simulink model "EngineModel_scaled_27_7_2016_with_new_maps"  (R2021a)
settings: Solver=ode4  StartTime=0.0  StopTime=30  FixedStep=0.2  RelTol=1e-3  EnableMultiTasking=on
values from neighbouring files (symbols this model uses):
  Fanmap_2 = [1 1 1 1 1 1 1 1 1 1 275.724 325.4224 ... (330 elements, 10x3x11)]    [enginemaps2.mat]
  HPCompmap_2 = [1 1 1 1 1 1 1 1 1 1 32.390865 37.6623195 ... (330 elements, 10x3x11)]    [enginemaps2.mat]
  HPTurbinemap_2 = [0.24979968 0.24979968 0.24979968 0.24979968 0.24979968 0.24979968 0.24979968 0.24979968 0.24979968 0.24979968 0.004250667 0.005047667 ... (330 elements, 10x3x11)]    [enginemaps2.mat]
  LPCompmap_2 = [1 1 1 1 1 1 1 1 1 1 34.17260994 40.23277722 ... (330 elements, 10x3x11)]    [enginemaps2.mat]
  LPTurbinemap_2 = [0.665969797 0.665969797 0.665969797 0.665969797 0.665969797 0.665969797 0.665969797 0.665969797 0.00912 0.013173333 0.015706667 0.01672 ... (264 elements, 8x3x11)]    [enginemaps2.mat]
undefined symbols (not defined in the file or in its folder): Adiabatic_compression_fan, Adiabatic_compression_HPC, Adiabatic_compression_LPC, coldnozzle, compression_ram, cond_f2, D, datatables, hotnozzle, HPT1, if_Nth, if_Ntl, if_Z, LPT, performance1, thermo_combustor, turbo
libraries: dspmtrx3 x10, aerolibatmos2 x8, dspsigattribs x3, dspsolvers x2, dspfactors x1
(part 9 of 14)

== system EngineModel_scaled_27_7_2016_with_new_maps/Double spool TFE CF6-50 steady state modeling (BOING 747-200)/Error Due to Vs/Error Due To Dv7/HPT/ HP turbine ==
  Pt45 : Inport
  Cp45_old : Inport  Port=2
  F_A : Inport  Port=3
  Ht45_old : Inport  Port=4
  Wg4 : Inport  Port=5
  Wg45 : Inport  Port=6
  wach : Inport  Port=7
  Ht3 : Inport  Port=8
  Demux : Demux  Outputs=5
      settings: DisplayOption=none
  Interpreted MATLAB Function : MATLABFcn  MATLABFcn=turbo (u(1),u(2),u(3),u(4),u(5),u(6),u(7),u(8))  OutputDimensions=5
  Mux : Mux  Inputs=8
      settings: DisplayOption=signals
  Cp45 : Outport
  Tt45 : Outport  Port=2
  S45 : Outport  Port=3
  Ht45 : Outport  Port=4
  F/A : Outport  Port=5
  wires:
  Mux/1 -> Interpreted MATLAB Function/1
  Interpreted MATLAB Function/1 -> Demux/1
  Pt45/1 -> Mux/1
  Cp45_old/1 -> Mux/2
  F_A/1 -> Mux/3
  Ht45_old/1 -> Mux/4
  Wg4/1 -> Mux/5
  Wg45/1 -> Mux/6
  wach/1 -> Mux/7
  Ht3/1 -> Mux/8
  Demux/1 -> Cp45/1
  Demux/2 -> Tt45/1
  Demux/3 -> S45/1
  Demux/4 -> Ht45/1
  Demux/5 -> F/A/1

== system EngineModel_scaled_27_7_2016_with_new_maps/Double spool TFE CF6-50 steady state modeling (BOING 747-200)/Error Due to Vs/Error Due To Dv7/HPT/enthalpy_MAPS ==
  Ht4 : Inport
  Tt4 : Inport  Port=2
  Tt2.5 : Inport  Port=3
  Nch : Inport  Port=4
  TFth : Inport  Port=5
  " \"unit conversion\"" : Constant  Value=4.184
  Display{1..7} (7 alike) : Display
  HPT map : Subsystem
  Nch_Nth : Subsystem
  Product1 : Product  Inputs=*/  SaturateOnIntegerOverflow=on  OutDataTypeStr=Inherit: Same as first input
  Product5 : Product  Inputs=***  SaturateOnIntegerOverflow=on  OutDataTypeStr=Inherit: Same as first input
  Sum : Sum  Inputs=-+  SaturateOnIntegerOverflow=on
  Sum1 : Sum  Inputs=-+  SaturateOnIntegerOverflow=on
  Ht45s : Outport
  (DH/T)th : Outport  Port=2
  Ht45_old : Outport  Port=3
  wires:
  Sum1/1 -> Display4/1, Ht45s/1
  Nch/1 -> Nch_Nth/3(Nch)
  Nch_Nth/1(Nth) -> HPT map/1(Nth), Display5/1
  TFth/1 -> HPT map/2(TFth)
  HPT map/1((DH/T)th) -> Product5/3, Display1/1, (DH/T)th/1
  Ht4/1 -> Display3/1, Sum/2, Sum1/2
  Product5/1 -> Display2/1, Sum/1, Product1/1
  HPT map/2(etath) -> Display6/1, Product1/2
  Product1/1 -> Sum1/1
  Tt4/1 -> Product5/2, Nch_Nth/1(Tt4)
  Tt2.5/1 -> Nch_Nth/2(Tt2.5)
  " \"unit conversion\""/1 -> Product5/1
  Sum/1 -> Display7/1, Ht45_old/1

== system EngineModel_scaled_27_7_2016_with_new_maps/Double spool TFE CF6-50 steady state modeling (BOING 747-200)/Error Due to Vs/Error Due To Dv7/HPT/thermo_turbine ==
  Ht45s : Inport
  Ht45_old : Inport  Port=2
  Pt4 : Inport  Port=3
  Cp4 : Inport  Port=4
  F/A : Inport  Port=5
  S4 : Inport  Port=6
  Demux : Demux
      settings: DisplayOption=none
  Interpreted MATLAB Function : MATLABFcn  MATLABFcn=HPT1 (u(1),u(2),u(3),u(4),u(5),u(6))  OutputDimensions=4
  Mux : Mux  Inputs=6
      settings: DisplayOption=signals
  Pt45 : Outport
  Tt45 : Outport  Port=2
  S45 : Outport  Port=3
  Cp45 : Outport  Port=4
  wires:
  Interpreted MATLAB Function/1 -> Demux/1
  Mux/1 -> Interpreted MATLAB Function/1
  Ht45s/1 -> Mux/1
  Ht45_old/1 -> Mux/2
  Pt4/1 -> Mux/3
  Cp4/1 -> Mux/4
  Demux/1 -> Pt45/1
  Demux/2 -> Tt45/1
  Demux/3 -> S45/1
  F/A/1 -> Mux/5
  S4/1 -> Mux/6
  Demux/4 -> Cp45/1

== system EngineModel_scaled_27_7_2016_with_new_maps/Double spool TFE CF6-50 steady state modeling (BOING 747-200)/Error Due to Vs/Error Due To Dv7/LPC/Adiabatic compression ==
  Tt13 : Inport  PortDimensions=1
  Pt13 : Inport  Port=2  PortDimensions=1
  Prcl : Inport  Port=3  PortDimensions=1
  etacl : Inport  Port=4  PortDimensions=1
  Ht13 : Inport  Port=5  PortDimensions=1
  S13 : Inport  Port=6  PortDimensions=1
  isentropic compression : Subsystem
  Tt25 : Outport
  Pt25 : Outport  Port=2
  Ht25 : Outport  Port=3
  S25 : Outport  Port=4
  wires:
  Tt13/1 -> isentropic compression/1(Tt13)
  Prcl/1 -> isentropic compression/2(Prcl)
  Pt13/1 -> isentropic compression/3(P13)
  Ht13/1 -> isentropic compression/4(Ht13)
  S13/1 -> isentropic compression/5(S13)
  etacl/1 -> isentropic compression/6(etacl)
  isentropic compression/2(Tt25) -> Tt25/1
  isentropic compression/3(Pt25) -> Pt25/1
  isentropic compression/4(Ht25) -> Ht25/1
  isentropic compression/1(S25) -> S25/1

== system EngineModel_scaled_27_7_2016_with_new_maps/Double spool TFE CF6-50 steady state modeling (BOING 747-200)/Error Due to Vs/Error Due To Dv7/LPC/LPC Map ==
  Zcl : Inport
  Ncf : Inport  Port=2
  Display : Display
  Display1 : Display
  If condition Zcl : Subsystem
  LPC Map Lookuptable efficiency : Subsystem
  LPC Map Lookuptable massflow : Subsystem
  LPC Map Lookuptable pressure ratio : Subsystem
  Prcl : Outport
  etacl : Outport  Port=2
  MFPcl : Outport  Port=3
  wires:
  Zcl/1 -> If condition Zcl/1(Zcli), Display1/1
  ? -> ?
  If condition Zcl/1(Zcl) -> Display/1, LPC Map Lookuptable pressure ratio/2(Zcl), LPC Map Lookuptable efficiency/2(Zcl), LPC Map Lookuptable massflow/2(Zcl)
  Ncf/1 -> LPC Map Lookuptable pressure ratio/1(corr Speed Ncl), LPC Map Lookuptable efficiency/1(corr Speed Ncl), LPC Map Lookuptable massflow/1(corr Speed Ncl)
  LPC Map Lookuptable massflow/1(" MFPcl") -> MFPcl/1
  LPC Map Lookuptable efficiency/1(etacl) -> etacl/1
  LPC Map Lookuptable pressure ratio/1(" Prcl") -> Prcl/1

== system EngineModel_scaled_27_7_2016_with_new_maps/Double spool TFE CF6-50 steady state modeling (BOING 747-200)/Error Due to Vs/Error Due To Dv7/LPT/enthalpy_MAPS ==
  Ht45 : Inport
  Tt45 : Inport  Port=2
  Tt2 : Inport  Port=3
  Ncf : Inport  Port=4
  TFtl : Inport  Port=5
  " \"unit conversion\"" : Constant  Value=4.184
  Display{1..7} (7 alike) : Display
  LPT map : Subsystem
  Nch_Nth : Subsystem
  Product1 : Product  Inputs=*/  SaturateOnIntegerOverflow=on  OutDataTypeStr=Inherit: Same as first input
  Product5 : Product  Inputs=***  SaturateOnIntegerOverflow=on  OutDataTypeStr=Inherit: Same as first input
  Sum : Sum  Inputs=-+  SaturateOnIntegerOverflow=on
  Sum1 : Sum  Inputs=-+  SaturateOnIntegerOverflow=on
  Ht5s : Outport
  (DH/T)tl : Outport  Port=2
  Ht5 : Outport  Port=3
  wires:
  Sum1/1 -> Display4/1, Ht5s/1
  Ncf/1 -> Nch_Nth/3(Ncf)
  Nch_Nth/1(Ntl) -> LPT map/1(Ntl), Display5/1
  TFtl/1 -> LPT map/2(TFtl)
  LPT map/1((DH/T)tl) -> Product5/3, Display1/1, (DH/T)tl/1
  Ht45/1 -> Display3/1, Sum/2, Sum1/2
  Product5/1 -> Display2/1, Sum/1, Product1/1
  LPT map/2(etatl) -> Display6/1, Product1/2
  Product1/1 -> Sum1/1
  Tt45/1 -> Product5/2, Nch_Nth/1(Tt45)
  Tt2/1 -> Nch_Nth/2(Tt2)
  " \"unit conversion\""/1 -> Product5/1
  Sum/1 -> Display7/1, Ht5/1

== system EngineModel_scaled_27_7_2016_with_new_maps/Double spool TFE CF6-50 steady state modeling (BOING 747-200)/Error Due to Vs/Error Due To Dv7/LPT/thermo_turbine ==
  Ht5s : Inport
  Ht5 : Inport  Port=2
  Pt45 : Inport  Port=3
  Cp45 : Inport  Port=4
  F/A : Inport  Port=5
  S45 : Inport  Port=6
  Demux : Demux  Outputs=6
      settings: DisplayOption=none
  Interpreted MATLAB Function : MATLABFcn  MATLABFcn=LPT(u(1),u(2),u(3),u(4),u(5),u(6))  OutputDimensions=6
  Mux : Mux  Inputs=6
      settings: DisplayOption=signals
  Pt5 : Outport
  Tt5 : Outport  Port=2
  S5 : Outport  Port=3
  Cp5 : Outport  Port=4
  Gamma5 : Outport  Port=5
  Mw5 : Outport  Port=6
  wires:
  Interpreted MATLAB Function/1 -> Demux/1
  Mux/1 -> Interpreted MATLAB Function/1
  Ht5s/1 -> Mux/1
  Ht5/1 -> Mux/2
  Pt45/1 -> Mux/3
  Cp45/1 -> Mux/4
  Demux/1 -> Pt5/1
  Demux/2 -> Tt5/1
  Demux/3 -> S5/1
  F/A/1 -> Mux/5
  S45/1 -> Mux/6
  Demux/4 -> Cp5/1
  Demux/5 -> Gamma5/1
  Demux/6 -> Mw5/1

== system EngineModel_scaled_27_7_2016_with_new_maps/Double spool TFE CF6-50 steady state modeling (BOING 747-200)/Error Due to Vs/Error Due To Dv7/Ram/If condition PRF ==
  Mo : Inport
  Constant1 : Constant
  Constant2 : Constant  Value=1.35
  Constant3 : Constant  Value=0.075
  Constant4 : Constant  Value=935
  Constant5 : Constant  Value=800
  Display : Display
  Display1 : Display
  Display2 : Display
  Divide : Product  Inputs=*/
  If : If  IfExpression=u1 <1  ElseIfExpressions=u1>5  ZeroCross=off
  If Action Subsystem : Subsystem  TreatAsAtomicUnit=on
  If Action Subsystem1 : Subsystem  TreatAsAtomicUnit=on
  If Action Subsystem2 : Subsystem  TreatAsAtomicUnit=on
  Math Function1 : Math  Operator=pow  SignedPower=on  SaturateOnIntegerOverflow=on
  Math Function2 : Math  Operator=square  SignedPower=on  SaturateOnIntegerOverflow=on
  Math Function3 : Math  Operator=square  SignedPower=on  SaturateOnIntegerOverflow=on
  Matrix 1-Norm : dspmtrx3/Matrix  1-Norm  roundingMode=Floor  overflowMode=off  outputDataTypeStr=Inherit: Same as accumulator  outputMin=[]  outputMax=[]  outputLastDataTypeStr=Inherit: Same as accumulator
      settings: SourceProductBaseCode=DS
  Mux : Mux  Inputs=3
  Product7 : Product
  Subtract2 : Sum  Inputs=+-
  Subtract3 : Sum  Inputs=+-
  add : Sum
  etar : Outport
  wires:
  Subtract3/1 -> If Action Subsystem1/1(In1)
  Mux/1 -> Matrix 1-Norm/1
  Math Function1/1 -> Product7/1
  Product7/1 -> Subtract3/2
  Constant2/1 -> Math Function1/2
  If Action Subsystem/1(Out1) -> Mux/1, Display/1
  Subtract2/1 -> Math Function1/1
  Constant3/1 -> Product7/2
  Constant1/1 -> Subtract2/2, Subtract3/1, If Action Subsystem/1(In1)
  Math Function2/1 -> add/1
  Constant4/1 -> add/2
  Constant5/1 -> Divide/1
  add/1 -> Divide/2
  Divide/1 -> If Action Subsystem2/1(In1)
  Mo/1 -> Subtract2/1, If/1, Math Function3/1
  Math Function3/1 -> Math Function2/1
  If/1 -> If Action Subsystem/Action
  If/3 -> If Action Subsystem1/Action
  If/2 -> If Action Subsystem2/Action
  If Action Subsystem2/1(Out1) -> Mux/2, Display2/1
  If Action Subsystem1/1(Out1) -> Display1/1, Mux/3
  Matrix 1-Norm/1 -> etar/1

== system EngineModel_scaled_27_7_2016_with_new_maps/Double spool TFE CF6-50 steady state modeling (BOING 747-200)/Error Due to Vs/Error Due To Dv7/Ram/Ram compression ==
  Tt2 : Inport
  Pt2 : Inport  Port=2
  Demux : Demux  Outputs=3
      settings: DisplayOption=none
  Interpreted MATLAB Function : MATLABFcn  MATLABFcn=compression_ram(u(1),u(2))  OutputDimensions=3
  Mux : Mux  Inputs=2
      settings: DisplayOption=signals
  Ht2 : Outport
  S2 : Outport  Port=2
  Cp2 : Outport  Port=3
  wires:
  Tt2/1 -> Mux/1
  Interpreted MATLAB Function/1 -> Demux/1
  Mux/1 -> Interpreted MATLAB Function/1
  Pt2/1 -> Mux/2
  Demux/1 -> Ht2/1
  Demux/2 -> S2/1
  Demux/3 -> Cp2/1

== system EngineModel_scaled_27_7_2016_with_new_maps/Double spool TFE CF6-50 steady state modeling (BOING 747-200)/Off- Design Module/Combustor/Thermo_combustor/Combustor thermo ==
  Pt4 : Inport
  Ht4 : Inport  Port=2
  F/A : Inport  Port=3
  Cp3 : Inport  Port=4
  Demux : Demux
      settings: DisplayOption=none
  Interpreted MATLAB Function : MATLABFcn  MATLABFcn=thermo_combustor(u(1),u(2),u(3),u(4))  OutputDimensions=4
  Mux : Mux
      settings: DisplayOption=signals
  Tt4 : Outport
  S4 : Outport  Port=2
  Cp4 : Outport  Port=3
  Mw4 : Outport  Port=4
  wires:
  Mux/1 -> Interpreted MATLAB Function/1
  Interpreted MATLAB Function/1 -> Demux/1
  Ht4/1 -> Mux/2
  Pt4/1 -> Mux/1
  F/A/1 -> Mux/3
  Demux/1 -> Tt4/1
  Demux/2 -> S4/1
  Demux/3 -> Cp4/1
  Demux/4 -> Mw4/1
  Cp3/1 -> Mux/4

== system EngineModel_scaled_27_7_2016_with_new_maps/Double spool TFE CF6-50 steady state modeling (BOING 747-200)/Off- Design Module/Combustor/combustor o//p pressure/If Action Subsystem ==
  In1 : Inport
  Action Port : ActionPort  ActionPortLabel=if(u1 > 1)
  Out1 : Outport
  wires:
  In1/1 -> Out1/1

== system EngineModel_scaled_27_7_2016_with_new_maps/Double spool TFE CF6-50 steady state modeling (BOING 747-200)/Off- Design Module/Combustor/combustor o//p pressure/If Action Subsystem1 ==
  In1 : Inport
  Action Port : ActionPort  ActionPortLabel=else
  Out1 : Outport
  wires:
  In1/1 -> Out1/1

== system EngineModel_scaled_27_7_2016_with_new_maps/Double spool TFE CF6-50 steady state modeling (BOING 747-200)/Off- Design Module/Fan/Adiabatic compression/isentropic compression ==
  Tt2 : Inport
  Pr : Inport  Port=2
  Pt2 : Inport  Port=3
  Ht2 : Inport  Port=4
  S2 : Inport  Port=5
  etaf : Inport  Port=6
  Demux : Demux
      settings: DisplayOption=none
  Interpreted MATLAB Function : MATLABFcn  MATLABFcn=Adiabatic_compression_fan(u(1),u(2),u(3),u(4),u(5),u(6))  OutputDimensions=4
  Mux : Mux  Inputs=6
      settings: DisplayOption=signals
  S13 : Outport
  Tt13 : Outport  Port=2
  Pt13 : Outport  Port=3
  Ht13 : Outport  Port=4
  wires:
  Tt2/1 -> Mux/1
  Demux/2 -> Pt13/1
  Interpreted MATLAB Function/1 -> Demux/1
  Demux/1 -> Tt13/1
  Mux/1 -> Interpreted MATLAB Function/1
  Pt2/1 -> Mux/3
  Pr/1 -> Mux/2
  Ht2/1 -> Mux/4
  S2/1 -> Mux/5
  Demux/3 -> S13/1
  etaf/1 -> Mux/6
  Demux/4 -> Ht13/1

== system EngineModel_scaled_27_7_2016_with_new_maps/Double spool TFE CF6-50 steady state modeling (BOING 747-200)/Off- Design Module/Fan/Fan Map/Fan Map Lookuptable mass flow ==
  Ncf : Inport
  Zf : Inport  Port=2
  Constant : Constant  Value=2
  Display : Display
  massflow 3D fanmap Lookup Table : Lookup_n-D  NumberOfTableDimensions=3  BreakpointsForDimension1=[0.3,0.4,0.5,0.6,0.7,0.8,0.9,1.0,1.1,1.2]  BreakpointsForDimension2=[1,2,3]  BreakpointsForDimension3=[0,0.1,0.2,0.3,0.4,0.5,0.6,0.7,0.8,0.9,1]  IndexSearchMethod=Linear search  Table=Fanmap_2  InterpMethod=Cubic spline  ExtrapMethod=Cubic spline  OutDataTypeStr=double  RndMeth=Simplest
      settings: InputPortMap=u0,u1,u2
  Fan MFPf : Outport
  wires:
  massflow 3D fanmap Lookup Table/1 -> Fan MFPf/1, Display/1
  Constant/1 -> massflow 3D fanmap Lookup Table/2
  Ncf/1 -> massflow 3D fanmap Lookup Table/1
  Zf/1 -> massflow 3D fanmap Lookup Table/3

== system EngineModel_scaled_27_7_2016_with_new_maps/Double spool TFE CF6-50 steady state modeling (BOING 747-200)/Off- Design Module/Fan/Fan Map/Fan Map Lookuptable efficiency ==
  Ncf : Inport
  Zf : Inport  Port=2
  Constant : Constant  Value=3
  Display : Display
  massflow 3D fanmap Lookup Table : Lookup_n-D  NumberOfTableDimensions=3  BreakpointsForDimension1=[0.3,0.4,0.5,0.6,0.7,0.8,0.9,1.0,1.1,1.2]  BreakpointsForDimension2=[1,2,3]  BreakpointsForDimension3=[0,0.1,0.2,0.3,0.4,0.5,0.6,0.7,0.8,0.9,1]  IndexSearchMethod=Linear search  Table=Fanmap_2  InterpMethod=Cubic spline  ExtrapMethod=Cubic spline  OutDataTypeStr=double  RndMeth=Simplest
      settings: InputPortMap=u0,u1,u2
  Fan etaf : Outport
  wires:
  massflow 3D fanmap Lookup Table/1 -> Fan etaf/1, Display/1
  Constant/1 -> massflow 3D fanmap Lookup Table/2
  Ncf/1 -> massflow 3D fanmap Lookup Table/1
  Zf/1 -> massflow 3D fanmap Lookup Table/3

== system EngineModel_scaled_27_7_2016_with_new_maps/Double spool TFE CF6-50 steady state modeling (BOING 747-200)/Off- Design Module/Fan/Fan Map/Fan Map Lookuptable pressure ratio ==
  Ncf : Inport
  Zf : Inport  Port=2
  Constant : Constant
  Display : Display
  massflow 3D fanmap Lookup Table : Lookup_n-D  NumberOfTableDimensions=3  BreakpointsForDimension1=[0.3,0.4,0.5,0.6,0.7,0.8,0.9,1.0,1.1,1.2]  BreakpointsForDimension2=[1,2,3]  BreakpointsForDimension3=[0,0.1,0.2,0.3,0.4,0.5,0.6,0.7,0.8,0.9,1]  IndexSearchMethod=Linear search  Table=Fanmap_2  InterpMethod=Cubic spline  ExtrapMethod=Cubic spline  OutDataTypeStr=double  RndMeth=Simplest
      settings: InputPortMap=u0,u1,u2
  Fan Prf : Outport
  wires:
  Zf/1 -> massflow 3D fanmap Lookup Table/3
  Ncf/1 -> massflow 3D fanmap Lookup Table/1
  Constant/1 -> massflow 3D fanmap Lookup Table/2
  massflow 3D fanmap Lookup Table/1 -> Display/1, Fan Prf/1

== system EngineModel_scaled_27_7_2016_with_new_maps/Double spool TFE CF6-50 steady state modeling (BOING 747-200)/Off- Design Module/Fan/Fan Map/If condition Zf ==
  Zfi : Inport
  Demux : Demux  Outputs=1
      settings: DisplayOption=none
  Interpreted MATLAB Function : MATLABFcn  MATLABFcn=if_Z(u(1))  OutputDimensions=1
  Mux : Mux  Inputs=1
      settings: DisplayOption=signals
  Zf : Outport
  wires:
  Interpreted MATLAB Function/1 -> Demux/1
  Mux/1 -> Interpreted MATLAB Function/1
  Demux/1 -> Zf/1
  Zfi/1 -> Mux/1

== system EngineModel_scaled_27_7_2016_with_new_maps/Double spool TFE CF6-50 steady state modeling (BOING 747-200)/Off- Design Module/HPC/Adiabatic compression/isentropic compression ==
  Tt25 : Inport
  Prcl : Inport  Port=2
  Pt25 : Inport  Port=3
  Ht25 : Inport  Port=4
  S25 : Inport  Port=5
  etacl : Inport  Port=6
  Demux : Demux  Outputs=5
      settings: DisplayOption=none
  Display : Display
  Interpreted MATLAB Function : MATLABFcn  MATLABFcn=Adiabatic_compression_HPC(u(1),u(2),u(3),u(4),u(5),u(6))  OutputDimensions=5
  Mux : Mux  Inputs=6
      settings: DisplayOption=signals
  Tt3 : Outport
  Pt3 : Outport  Port=2
  S3 : Outport  Port=3
  Ht3 : Outport  Port=4
  Cp3 : Outport  Port=5
  wires:
  Tt25/1 -> Mux/1
  Demux/2 -> Pt3/1
  Interpreted MATLAB Function/1 -> Demux/1
  Demux/1 -> Display/1, Tt3/1
  Mux/1 -> Interpreted MATLAB Function/1
  Pt25/1 -> Mux/3
  Prcl/1 -> Mux/2
  Ht25/1 -> Mux/4
  S25/1 -> Mux/5
  Demux/3 -> S3/1
  etacl/1 -> Mux/6
  Demux/4 -> Ht3/1
  Demux/5 -> Cp3/1

== system EngineModel_scaled_27_7_2016_with_new_maps/Double spool TFE CF6-50 steady state modeling (BOING 747-200)/Off- Design Module/HPC/HPC Map/HPComp Map Lookup Table Massflow ==
  Corr Speed Nch : Inport
  zch : Inport  Port=2
  3D HPC map Lookup Table massflow : Lookup_n-D  NumberOfTableDimensions=3  BreakpointsForDimension1=[0.562,0.674,0.787,0.899,1,1.034,1.067,1.124,1.236,1.292]  BreakpointsForDimension2=[1,2,3]  BreakpointsForDimension3=[0,0.1,0.2,0.3,0.4,0.5,0.6,0.7,0.8,0.9,1]  IndexSearchMethod=Linear search  Table=HPCompmap_2  InterpMethod=Cubic spline  ExtrapMethod=Cubic spline  OutDataTypeStr=double  RndMeth=Simplest
      settings: InputPortMap=u0,u1,u2
  Constant1 : Constant  Value=2
  Display : Display
  HPC MFPch : Outport
  wires:
  Constant1/1 -> 3D HPC map Lookup Table massflow/2
  Corr Speed Nch/1 -> 3D HPC map Lookup Table massflow/1
  3D HPC map Lookup Table massflow/1 -> HPC MFPch/1, Display/1
  zch/1 -> 3D HPC map Lookup Table massflow/3

== system EngineModel_scaled_27_7_2016_with_new_maps/Double spool TFE CF6-50 steady state modeling (BOING 747-200)/Off- Design Module/HPC/HPC Map/HPComp Map Lookup Table efficiency ==
  Corr Speed Nch : Inport
  zch : Inport  Port=2
  3D HPC map Lookup Table efficiency : Lookup_n-D  NumberOfTableDimensions=3  BreakpointsForDimension1=[0.562,0.674,0.787,0.899,1,1.034,1.067,1.124,1.236,1.292]  BreakpointsForDimension2=[1,2,3]  BreakpointsForDimension3=[0,0.1,0.2,0.3,0.4,0.5,0.6,0.7,0.8,0.9,1]  IndexSearchMethod=Linear search  Table=HPCompmap_2  InterpMethod=Cubic spline  ExtrapMethod=Cubic spline  OutDataTypeStr=double  RndMeth=Simplest
      settings: InputPortMap=u0,u1,u2
  Constant1 : Constant  Value=3
  Display : Display
  HPC etach : Outport
  wires:
  Constant1/1 -> 3D HPC map Lookup Table efficiency/2
  Corr Speed Nch/1 -> 3D HPC map Lookup Table efficiency/1
  3D HPC map Lookup Table efficiency/1 -> HPC etach/1, Display/1
  zch/1 -> 3D HPC map Lookup Table efficiency/3

== system EngineModel_scaled_27_7_2016_with_new_maps/Double spool TFE CF6-50 steady state modeling (BOING 747-200)/Off- Design Module/HPC/HPC Map/HPComp Map Lookup Table pressure ratio ==
  Corr Speed Nch : Inport
  zch : Inport  Port=2
  3D HPC map Lookup Table pressure ratio : Lookup_n-D  NumberOfTableDimensions=3  BreakpointsForDimension1=[0.562,0.674,0.787,0.899,1,1.034,1.067,1.124,1.236,1.292]  BreakpointsForDimension2=[1,2,3]  BreakpointsForDimension3=[0,0.1,0.2,0.3,0.4,0.5,0.6,0.7,0.8,0.9,1]  IndexSearchMethod=Linear search  Table=HPCompmap_2  InterpMethod=Cubic spline  ExtrapMethod=Cubic spline  OutDataTypeStr=double  RndMeth=Simplest
      settings: InputPortMap=u0,u1,u2
  Constant1 : Constant
  Display : Display
  HPC Prch : Outport
  wires:
  zch/1 -> 3D HPC map Lookup Table pressure ratio/3
  3D HPC map Lookup Table pressure ratio/1 -> Display/1, HPC Prch/1
  Corr Speed Nch/1 -> 3D HPC map Lookup Table pressure ratio/1
  Constant1/1 -> 3D HPC map Lookup Table pressure ratio/2

== system EngineModel_scaled_27_7_2016_with_new_maps/Double spool TFE CF6-50 steady state modeling (BOING 747-200)/Off- Design Module/HPC/HPC Map/If condition Zf ==
  Zchi : Inport
  Demux : Demux  Outputs=1
      settings: DisplayOption=none
  Interpreted MATLAB Function : MATLABFcn  MATLABFcn=if_Z(u(1))  OutputDimensions=1
  Mux : Mux  Inputs=1
      settings: DisplayOption=signals
  Zch : Outport
  wires:
  Interpreted MATLAB Function/1 -> Demux/1
  Mux/1 -> Interpreted MATLAB Function/1
  Demux/1 -> Zch/1
  Zchi/1 -> Mux/1

== system EngineModel_scaled_27_7_2016_with_new_maps/Double spool TFE CF6-50 steady state modeling (BOING 747-200)/Off- Design Module/HPT/enthalpy_MAPS/HPT map ==
  Nth : Inport
  TFth : Inport  Port=2
  HPT Map lookup Table (DH/T) : Subsystem
  HPT Map lookup Table Efficency : Subsystem
  (DH/T)th : Outport
  etath : Outport  Port=2
  wires:
  Nth/1 -> HPT Map lookup Table Efficency/1(corr speed Nth), HPT Map lookup Table (DH/T)/1(corr speed Nth)
  TFth/1 -> HPT Map lookup Table Efficency/2(TFth), HPT Map lookup Table (DH/T)/2(TFth)
  HPT Map lookup Table (DH/T)/1(HPT (DH/T)th) -> (DH/T)th/1
  HPT Map lookup Table Efficency/1(HPT Ettath) -> etath/1

== system EngineModel_scaled_27_7_2016_with_new_maps/Double spool TFE CF6-50 steady state modeling (BOING 747-200)/Off- Design Module/HPT/enthalpy_MAPS/Nch_Nth ==
  Tt4 : Inport
  Tt2.5 : Inport  Port=2
  Nch : Inport  Port=3
  (To)Ref : Constant  Value=288
  (theta4)d : Constant  Value=1.1018
  Display5 : Display
  Product3 : Product  Inputs=***  SaturateOnIntegerOverflow=on  OutDataTypeStr=Inherit: Same as first input
  Product4 : Product  Inputs=*/  SaturateOnIntegerOverflow=on  OutDataTypeStr=Inherit: Same as first input
  Product6 : Product  Inputs=*/  SaturateOnIntegerOverflow=on  OutDataTypeStr=Inherit: Same as first input
  Product7 : Product  Inputs=*/  SaturateOnIntegerOverflow=on  OutDataTypeStr=Inherit: Same as first input
  Sqrt1 : Sqrt  SaturateOnIntegerOverflow=on
  Sqrt2 : Sqrt  SaturateOnIntegerOverflow=on
  const. : Constant  Value=100
  Nth : Outport
  wires:
  Product7/1 -> Product3/1
  (To)Ref/1 -> Product4/2
  Sqrt1/1 -> Product7/2
  const./1 -> Product7/1
  Product3/1 -> Nth/1, Display5/1
  Tt4/1 -> Sqrt1/1
  Tt2.5/1 -> Product4/1
  Product4/1 -> Sqrt2/1
  (theta4)d/1 -> Product6/2
  Product6/1 -> Product3/2
  Sqrt2/1 -> Product6/1
  Nch/1 -> Product3/3

== system EngineModel_scaled_27_7_2016_with_new_maps/Double spool TFE CF6-50 steady state modeling (BOING 747-200)/Off- Design Module/LPC/Adiabatic compression/isentropic compression ==
  Tt13 : Inport
  Prcl : Inport  Port=2
  P13 : Inport  Port=3
  Ht13 : Inport  Port=4
  S13 : Inport  Port=5
  etacl : Inport  Port=6
  Demux : Demux
      settings: DisplayOption=none
  Interpreted MATLAB Function : MATLABFcn  MATLABFcn=Adiabatic_compression_LPC(u(1),u(2),u(3),u(4),u(5),u(6))  OutputDimensions=4
  Mux : Mux  Inputs=6
      settings: DisplayOption=signals
  S25 : Outport
  Tt25 : Outport  Port=2
  Pt25 : Outport  Port=3
  Ht25 : Outport  Port=4
  wires:
  Tt13/1 -> Mux/1
  Demux/2 -> Pt25/1
  Interpreted MATLAB Function/1 -> Demux/1
  Demux/1 -> Tt25/1
  Mux/1 -> Interpreted MATLAB Function/1
  P13/1 -> Mux/3
  Prcl/1 -> Mux/2
  Ht13/1 -> Mux/4
  S13/1 -> Mux/5
  Demux/3 -> S25/1
  etacl/1 -> Mux/6
  Demux/4 -> Ht25/1

== system EngineModel_scaled_27_7_2016_with_new_maps/Double spool TFE CF6-50 steady state modeling (BOING 747-200)/Off- Design Module/LPC/LPC Map/If condition Zf ==
  Zcli : Inport
  Demux : Demux  Outputs=1
      settings: DisplayOption=none
  Interpreted MATLAB Function : MATLABFcn  MATLABFcn=if_Z(u(1))  OutputDimensions=1
  Mux : Mux  Inputs=1
      settings: DisplayOption=signals
  Zcl : Outport
  wires:
  Interpreted MATLAB Function/1 -> Demux/1
  Mux/1 -> Interpreted MATLAB Function/1
  Demux/1 -> Zcl/1
  Zcli/1 -> Mux/1

== system EngineModel_scaled_27_7_2016_with_new_maps/Double spool TFE CF6-50 steady state modeling (BOING 747-200)/Off- Design Module/LPC/LPC Map/LPC Map Lookuptable efficiency ==
  corr Speed Ncl : Inport
  Zcl : Inport  Port=2
  3D fanmap Lookup Table : Lookup_n-D  NumberOfTableDimensions=3  BreakpointsForDimension1=[0.3,0.4,0.5,0.6,0.7,0.8,0.9,1.0,1.1,1.2]  BreakpointsForDimension2=[1,2,3]  BreakpointsForDimension3=[0,0.1,0.2,0.3,0.4,0.5,0.6,0.7,0.8,0.9,1]  IndexSearchMethod=Linear search  Table=LPCompmap_2  InterpMethod=Cubic spline  ExtrapMethod=Cubic spline  OutDataTypeStr=double  RndMeth=Simplest
      settings: InputPortMap=u0,u1,u2
  Constant1 : Constant  Value=3
  Display : Display
  etacl : Outport
  wires:
  corr Speed Ncl/1 -> 3D fanmap Lookup Table/1
  Constant1/1 -> 3D fanmap Lookup Table/2
  3D fanmap Lookup Table/1 -> etacl/1, Display/1
  Zcl/1 -> 3D fanmap Lookup Table/3

== system EngineModel_scaled_27_7_2016_with_new_maps/Double spool TFE CF6-50 steady state modeling (BOING 747-200)/Off- Design Module/LPC/LPC Map/LPC Map Lookuptable massflow ==
  corr Speed Ncl : Inport
  Zcl : Inport  Port=2
  3D fanmap Lookup Table : Lookup_n-D  NumberOfTableDimensions=3  BreakpointsForDimension1=[0.3,0.4,0.5,0.6,0.7,0.8,0.9,1.0,1.1,1.2]  BreakpointsForDimension2=[1,2,3]  BreakpointsForDimension3=[0,0.1,0.2,0.3,0.4,0.5,0.6,0.7,0.8,0.9,1]  IndexSearchMethod=Linear search  Table=LPCompmap_2  InterpMethod=Cubic spline  ExtrapMethod=Cubic spline  OutDataTypeStr=double  RndMeth=Simplest
      settings: InputPortMap=u0,u1,u2
  Constant1 : Constant  Value=2
  Display : Display
  " MFPcl" : Outport
  wires:
  corr Speed Ncl/1 -> 3D fanmap Lookup Table/1
  Constant1/1 -> 3D fanmap Lookup Table/2
  3D fanmap Lookup Table/1 -> " MFPcl"/1, Display/1
  Zcl/1 -> 3D fanmap Lookup Table/3

== system EngineModel_scaled_27_7_2016_with_new_maps/Double spool TFE CF6-50 steady state modeling (BOING 747-200)/Off- Design Module/LPC/LPC Map/LPC Map Lookuptable pressure ratio ==
  corr Speed Ncl : Inport
  Zcl : Inport  Port=2
  3D fanmap Lookup Table : Lookup_n-D  NumberOfTableDimensions=3  BreakpointsForDimension1=[0.3,0.4,0.5,0.6,0.7,0.8,0.9,1.0,1.1,1.2]  BreakpointsForDimension2=[1,2,3]  BreakpointsForDimension3=[0,0.1,0.2,0.3,0.4,0.5,0.6,0.7,0.8,0.9,1]  IndexSearchMethod=Linear search  Table=LPCompmap_2  InterpMethod=Cubic spline  ExtrapMethod=Cubic spline  OutDataTypeStr=double  RndMeth=Simplest
      settings: InputPortMap=u0,u1,u2
  Constant1 : Constant
  Display : Display
  " Prcl" : Outport
  wires:
  Zcl/1 -> 3D fanmap Lookup Table/3
  3D fanmap Lookup Table/1 -> Display/1, " Prcl"/1
  Constant1/1 -> 3D fanmap Lookup Table/2
  corr Speed Ncl/1 -> 3D fanmap Lookup Table/1

== system EngineModel_scaled_27_7_2016_with_new_maps/Double spool TFE CF6-50 steady state modeling (BOING 747-200)/Off- Design Module/LPT/enthalpy_MAPS/LPT map ==
  Ntl : Inport
  TFtl : Inport  Port=2
  LPT Map lookup Table (DH/T) : Subsystem
  LPT Map lookup Table Efficency : Subsystem
  (DH/T)tl : Outport
  etatl : Outport  Port=2
  wires:
  Ntl/1 -> LPT Map lookup Table Efficency/1(corr speed Ntl), LPT Map lookup Table (DH/T)/1(corr speed Ntl)
  TFtl/1 -> LPT Map lookup Table Efficency/2(TFtl), LPT Map lookup Table (DH/T)/2(TFtl)
  LPT Map lookup Table (DH/T)/1(LPT (DH/T)tl) -> (DH/T)tl/1
  LPT Map lookup Table Efficency/1(HPT Ettatl) -> etatl/1

== system EngineModel_scaled_27_7_2016_with_new_maps/Double spool TFE CF6-50 steady state modeling (BOING 747-200)/Off- Design Module/LPT/enthalpy_MAPS/Nch_Nth ==
  Tt45 : Inport
  Tt2 : Inport  Port=2
  Ncf : Inport  Port=3
  (To)Ref : Constant  Value=288
  (theta2)d : Constant  Value=0.9532186
  Display5 : Display
  Product3 : Product  Inputs=**  SaturateOnIntegerOverflow=on  OutDataTypeStr=Inherit: Same as first input
  Product4 : Product  Inputs=*/  SaturateOnIntegerOverflow=on  OutDataTypeStr=Inherit: Same as first input
  Product6 : Product  Inputs=*/  SaturateOnIntegerOverflow=on  OutDataTypeStr=Inherit: Same as first input
  Product7 : Product  Inputs=*/  SaturateOnIntegerOverflow=on  OutDataTypeStr=Inherit: Same as first input
  Product8 : Product  Inputs=**  SaturateOnIntegerOverflow=on  OutDataTypeStr=Inherit: Same as first input
  Sqrt1 : Sqrt  SaturateOnIntegerOverflow=on
  Sqrt2 : Sqrt  SaturateOnIntegerOverflow=on
  const. : Constant  Value=100
  Ntl : Outport
  wires:
  Product8/1 -> Product3/1
  (To)Ref/1 -> Product4/2
  Product7/1 -> Product8/1
  Sqrt1/1 -> Product7/2
  const./1 -> Product7/1
  Product3/1 -> Display5/1, Ntl/1
  Ncf/1 -> Product3/2
  Tt45/1 -> Sqrt1/1
  Tt2/1 -> Product4/1
  Product4/1 -> Sqrt2/1
  (theta2)d/1 -> Product6/2
  Product6/1 -> Product8/2
  Sqrt2/1 -> Product6/1

== system EngineModel_scaled_27_7_2016_with_new_maps/Double spool TFE CF6-50 steady state modeling (BOING 747-200)/Off- Design Module/Ram/If condition PRF/If Action Subsystem ==
  In1 : Inport
  Action Port : ActionPort  ActionPortLabel=if(u1 <1)
  Out1 : Outport
  wires:
  In1/1 -> Out1/1

== system EngineModel_scaled_27_7_2016_with_new_maps/Double spool TFE CF6-50 steady state modeling (BOING 747-200)/Off- Design Module/Ram/If condition PRF/If Action Subsystem1 ==
  In1 : Inport
  Action Port : ActionPort  ActionPortLabel=else
  Out1 : Outport
  wires:
  In1/1 -> Out1/1

== system EngineModel_scaled_27_7_2016_with_new_maps/Double spool TFE CF6-50 steady state modeling (BOING 747-200)/Off- Design Module/Ram/If condition PRF/If Action Subsystem2 ==
  In1 : Inport
  Action Port : ActionPort  ActionPortLabel=elseif(u1>5)
  Out1 : Outport
  wires:
  In1/1 -> Out1/1

== system EngineModel_scaled_27_7_2016_with_new_maps/Double spool TFE CF6-50 steady state modeling (BOING 747-200)/Error Due to Vs/Error Due To Dv1/Combustor/Thermo_combustor/Combustor thermo ==
  Pt4 : Inport
  Ht4 : Inport  Port=2
  F/A : Inport  Port=3
  Cp3 : Inport  Port=4
  Demux : Demux
      settings: DisplayOption=none
  Interpreted MATLAB Function : MATLABFcn  MATLABFcn=thermo_combustor(u(1),u(2),u(3),u(4))  OutputDimensions=4
  Mux : Mux
      settings: DisplayOption=signals
  Tt4 : Outport
  S4 : Outport  Port=2
  Cp4 : Outport  Port=3
  Mw4 : Outport  Port=4
  wires:
  Mux/1 -> Interpreted MATLAB Function/1
  Interpreted MATLAB Function/1 -> Demux/1
  Ht4/1 -> Mux/2
  Pt4/1 -> Mux/1
  F/A/1 -> Mux/3
  Demux/1 -> Tt4/1
  Demux/2 -> S4/1
  Demux/3 -> Cp4/1
  Demux/4 -> Mw4/1
  Cp3/1 -> Mux/4

== system EngineModel_scaled_27_7_2016_with_new_maps/Double spool TFE CF6-50 steady state modeling (BOING 747-200)/Error Due to Vs/Error Due To Dv1/Combustor/combustor o//p pressure/If Action Subsystem ==
  In1 : Inport
  Action Port : ActionPort  ActionPortLabel=if(u1 > 1)
  Out1 : Outport
  wires:
  In1/1 -> Out1/1

== system EngineModel_scaled_27_7_2016_with_new_maps/Double spool TFE CF6-50 steady state modeling (BOING 747-200)/Error Due to Vs/Error Due To Dv1/Combustor/combustor o//p pressure/If Action Subsystem1 ==
  In1 : Inport
  Action Port : ActionPort  ActionPortLabel=else
  Out1 : Outport
  wires:
  In1/1 -> Out1/1

== system EngineModel_scaled_27_7_2016_with_new_maps/Double spool TFE CF6-50 steady state modeling (BOING 747-200)/Error Due to Vs/Error Due To Dv1/Fan/Adiabatic compression/isentropic compression ==
  Tt2 : Inport
  Pr : Inport  Port=2
  Pt2 : Inport  Port=3
  Ht2 : Inport  Port=4
  S2 : Inport  Port=5
  etaf : Inport  Port=6
  Demux : Demux
      settings: DisplayOption=none
  Interpreted MATLAB Function : MATLABFcn  MATLABFcn=Adiabatic_compression_fan(u(1),u(2),u(3),u(4),u(5),u(6))  OutputDimensions=4
  Mux : Mux  Inputs=6
      settings: DisplayOption=signals
  S13 : Outport
  Tt13 : Outport  Port=2
  Pt13 : Outport  Port=3
  Ht13 : Outport  Port=4
  wires:
  Tt2/1 -> Mux/1
  Demux/2 -> Pt13/1
  Interpreted MATLAB Function/1 -> Demux/1
  Demux/1 -> Tt13/1
  Mux/1 -> Interpreted MATLAB Function/1
  Pt2/1 -> Mux/3
  Pr/1 -> Mux/2
  Ht2/1 -> Mux/4
  S2/1 -> Mux/5
  Demux/3 -> S13/1
  etaf/1 -> Mux/6
  Demux/4 -> Ht13/1

== system EngineModel_scaled_27_7_2016_with_new_maps/Double spool TFE CF6-50 steady state modeling (BOING 747-200)/Error Due to Vs/Error Due To Dv1/Fan/Fan Map/Fan Map Lookuptable mass flow ==
  Ncf : Inport
  Zf : Inport  Port=2
  Constant : Constant  Value=2
  Display : Display
  massflow 3D fanmap Lookup Table : Lookup_n-D  NumberOfTableDimensions=3  BreakpointsForDimension1=[0.3,0.4,0.5,0.6,0.7,0.8,0.9,1.0,1.1,1.2]  BreakpointsForDimension2=[1,2,3]  BreakpointsForDimension3=[0,0.1,0.2,0.3,0.4,0.5,0.6,0.7,0.8,0.9,1]  IndexSearchMethod=Linear search  Table=Fanmap_2  InterpMethod=Cubic spline  ExtrapMethod=Cubic spline  OutDataTypeStr=double  RndMeth=Simplest
      settings: InputPortMap=u0,u1,u2
  Fan MFPf : Outport
  wires:
  massflow 3D fanmap Lookup Table/1 -> Fan MFPf/1, Display/1
  Constant/1 -> massflow 3D fanmap Lookup Table/2
  Ncf/1 -> massflow 3D fanmap Lookup Table/1
  Zf/1 -> massflow 3D fanmap Lookup Table/3

== system EngineModel_scaled_27_7_2016_with_new_maps/Double spool TFE CF6-50 steady state modeling (BOING 747-200)/Error Due to Vs/Error Due To Dv1/Fan/Fan Map/Fan Map Lookuptable efficiency ==
  Ncf : Inport
  Zf : Inport  Port=2
  Constant : Constant  Value=3
  Display : Display
  massflow 3D fanmap Lookup Table : Lookup_n-D  NumberOfTableDimensions=3  BreakpointsForDimension1=[0.3,0.4,0.5,0.6,0.7,0.8,0.9,1.0,1.1,1.2]  BreakpointsForDimension2=[1,2,3]  BreakpointsForDimension3=[0,0.1,0.2,0.3,0.4,0.5,0.6,0.7,0.8,0.9,1]  IndexSearchMethod=Linear search  Table=Fanmap_2  InterpMethod=Cubic spline  ExtrapMethod=Cubic spline  OutDataTypeStr=double  RndMeth=Simplest
      settings: InputPortMap=u0,u1,u2
  Fan etaf : Outport
  wires:
  massflow 3D fanmap Lookup Table/1 -> Fan etaf/1, Display/1
  Constant/1 -> massflow 3D fanmap Lookup Table/2
  Ncf/1 -> massflow 3D fanmap Lookup Table/1
  Zf/1 -> massflow 3D fanmap Lookup Table/3

== system EngineModel_scaled_27_7_2016_with_new_maps/Double spool TFE CF6-50 steady state modeling (BOING 747-200)/Error Due to Vs/Error Due To Dv1/Fan/Fan Map/Fan Map Lookuptable pressure ratio ==
  Ncf : Inport
  Zf : Inport  Port=2
  Constant : Constant
  Display : Display
  massflow 3D fanmap Lookup Table : Lookup_n-D  NumberOfTableDimensions=3  BreakpointsForDimension1=[0.3,0.4,0.5,0.6,0.7,0.8,0.9,1.0,1.1,1.2]  BreakpointsForDimension2=[1,2,3]  BreakpointsForDimension3=[0,0.1,0.2,0.3,0.4,0.5,0.6,0.7,0.8,0.9,1]  IndexSearchMethod=Linear search  Table=Fanmap_2  InterpMethod=Cubic spline  ExtrapMethod=Cubic spline  OutDataTypeStr=double  RndMeth=Simplest
      settings: InputPortMap=u0,u1,u2
  Fan Prf : Outport
  wires:
  Zf/1 -> massflow 3D fanmap Lookup Table/3
  Ncf/1 -> massflow 3D fanmap Lookup Table/1
  Constant/1 -> massflow 3D fanmap Lookup Table/2
  massflow 3D fanmap Lookup Table/1 -> Display/1, Fan Prf/1

== system EngineModel_scaled_27_7_2016_with_new_maps/Double spool TFE CF6-50 steady state modeling (BOING 747-200)/Error Due to Vs/Error Due To Dv1/Fan/Fan Map/If condition Zf ==
  Zfi : Inport
  Demux : Demux  Outputs=1
      settings: DisplayOption=none
  Interpreted MATLAB Function : MATLABFcn  MATLABFcn=if_Z(u(1))  OutputDimensions=1
  Mux : Mux  Inputs=1
      settings: DisplayOption=signals
  Zf : Outport
  wires:
  Interpreted MATLAB Function/1 -> Demux/1
  Mux/1 -> Interpreted MATLAB Function/1
  Demux/1 -> Zf/1
  Zfi/1 -> Mux/1

== system EngineModel_scaled_27_7_2016_with_new_maps/Double spool TFE CF6-50 steady state modeling (BOING 747-200)/Error Due to Vs/Error Due To Dv1/HPC/Adiabatic compression/isentropic compression ==
  Tt25 : Inport
  Prcl : Inport  Port=2
  Pt25 : Inport  Port=3
  Ht25 : Inport  Port=4
  S25 : Inport  Port=5
  etacl : Inport  Port=6
  Demux : Demux  Outputs=5
      settings: DisplayOption=none
  Display : Display
  Interpreted MATLAB Function : MATLABFcn  MATLABFcn=Adiabatic_compression_HPC(u(1),u(2),u(3),u(4),u(5),u(6))  OutputDimensions=5
  Mux : Mux  Inputs=6
      settings: DisplayOption=signals
  Tt3 : Outport
  Pt3 : Outport  Port=2
  S3 : Outport  Port=3
  Ht3 : Outport  Port=4
  Cp3 : Outport  Port=5
  wires:
  Tt25/1 -> Mux/1
  Demux/2 -> Pt3/1
  Interpreted MATLAB Function/1 -> Demux/1
  Demux/1 -> Display/1, Tt3/1
  Mux/1 -> Interpreted MATLAB Function/1
  Pt25/1 -> Mux/3
  Prcl/1 -> Mux/2
  Ht25/1 -> Mux/4
  S25/1 -> Mux/5
  Demux/3 -> S3/1
  etacl/1 -> Mux/6
  Demux/4 -> Ht3/1
  Demux/5 -> Cp3/1

== system EngineModel_scaled_27_7_2016_with_new_maps/Double spool TFE CF6-50 steady state modeling (BOING 747-200)/Error Due to Vs/Error Due To Dv1/HPC/HPC Map/HPComp Map Lookup Table Massflow ==
  Corr Speed Nch : Inport
  zch : Inport  Port=2
  3D HPC map Lookup Table massflow : Lookup_n-D  NumberOfTableDimensions=3  BreakpointsForDimension1=[0.562,0.674,0.787,0.899,1,1.034,1.067,1.124,1.236,1.292]  BreakpointsForDimension2=[1,2,3]  BreakpointsForDimension3=[0,0.1,0.2,0.3,0.4,0.5,0.6,0.7,0.8,0.9,1]  IndexSearchMethod=Linear search  Table=HPCompmap_2  InterpMethod=Cubic spline  ExtrapMethod=Cubic spline  OutDataTypeStr=double  RndMeth=Simplest
      settings: InputPortMap=u0,u1,u2
  Constant1 : Constant  Value=2
  Display : Display
  HPC MFPch : Outport
  wires:
  Constant1/1 -> 3D HPC map Lookup Table massflow/2
  Corr Speed Nch/1 -> 3D HPC map Lookup Table massflow/1
  3D HPC map Lookup Table massflow/1 -> HPC MFPch/1, Display/1
  zch/1 -> 3D HPC map Lookup Table massflow/3

== system EngineModel_scaled_27_7_2016_with_new_maps/Double spool TFE CF6-50 steady state modeling (BOING 747-200)/Error Due to Vs/Error Due To Dv1/HPC/HPC Map/HPComp Map Lookup Table efficiency ==
  Corr Speed Nch : Inport
  zch : Inport  Port=2
  3D HPC map Lookup Table efficiency : Lookup_n-D  NumberOfTableDimensions=3  BreakpointsForDimension1=[0.562,0.674,0.787,0.899,1,1.034,1.067,1.124,1.236,1.292]  BreakpointsForDimension2=[1,2,3]  BreakpointsForDimension3=[0,0.1,0.2,0.3,0.4,0.5,0.6,0.7,0.8,0.9,1]  IndexSearchMethod=Linear search  Table=HPCompmap_2  InterpMethod=Cubic spline  ExtrapMethod=Cubic spline  OutDataTypeStr=double  RndMeth=Simplest
      settings: InputPortMap=u0,u1,u2
  Constant1 : Constant  Value=3
  Display : Display
  HPC etach : Outport
  wires:
  Constant1/1 -> 3D HPC map Lookup Table efficiency/2
  Corr Speed Nch/1 -> 3D HPC map Lookup Table efficiency/1
  3D HPC map Lookup Table efficiency/1 -> HPC etach/1, Display/1
  zch/1 -> 3D HPC map Lookup Table efficiency/3

== system EngineModel_scaled_27_7_2016_with_new_maps/Double spool TFE CF6-50 steady state modeling (BOING 747-200)/Error Due to Vs/Error Due To Dv1/HPC/HPC Map/HPComp Map Lookup Table pressure ratio ==
  Corr Speed Nch : Inport
  zch : Inport  Port=2
  3D HPC map Lookup Table pressure ratio : Lookup_n-D  NumberOfTableDimensions=3  BreakpointsForDimension1=[0.562,0.674,0.787,0.899,1,1.034,1.067,1.124,1.236,1.292]  BreakpointsForDimension2=[1,2,3]  BreakpointsForDimension3=[0,0.1,0.2,0.3,0.4,0.5,0.6,0.7,0.8,0.9,1]  IndexSearchMethod=Linear search  Table=HPCompmap_2  InterpMethod=Cubic spline  ExtrapMethod=Cubic spline  OutDataTypeStr=double  RndMeth=Simplest
      settings: InputPortMap=u0,u1,u2
  Constant1 : Constant
  Display : Display
  HPC Prch : Outport
  wires:
  zch/1 -> 3D HPC map Lookup Table pressure ratio/3
  3D HPC map Lookup Table pressure ratio/1 -> Display/1, HPC Prch/1
  Corr Speed Nch/1 -> 3D HPC map Lookup Table pressure ratio/1
  Constant1/1 -> 3D HPC map Lookup Table pressure ratio/2

== system EngineModel_scaled_27_7_2016_with_new_maps/Double spool TFE CF6-50 steady state modeling (BOING 747-200)/Error Due to Vs/Error Due To Dv1/HPC/HPC Map/If condition Zch ==
  Zchi : Inport
  Demux : Demux  Outputs=1
      settings: DisplayOption=none
  Interpreted MATLAB Function : MATLABFcn  MATLABFcn=if_Z(u(1))  OutputDimensions=1
  Mux : Mux  Inputs=1
      settings: DisplayOption=signals
  Zch : Outport
  wires:
  Interpreted MATLAB Function/1 -> Demux/1
  Mux/1 -> Interpreted MATLAB Function/1
  Demux/1 -> Zch/1
  Zchi/1 -> Mux/1

== system EngineModel_scaled_27_7_2016_with_new_maps/Double spool TFE CF6-50 steady state modeling (BOING 747-200)/Error Due to Vs/Error Due To Dv1/HPT/enthalpy_MAPS/HPT map ==
  Nth : Inport
  TFth : Inport  Port=2
  HPT Map lookup Table (DH/T) : Subsystem
  HPT Map lookup Table Efficency : Subsystem
  (DH/T)th : Outport
  etath : Outport  Port=2
  wires:
  Nth/1 -> HPT Map lookup Table Efficency/1(corr speed Nth), HPT Map lookup Table (DH/T)/1(corr speed Nth)
  TFth/1 -> HPT Map lookup Table Efficency/2(TFth), HPT Map lookup Table (DH/T)/2(TFth)
  HPT Map lookup Table (DH/T)/1(HPT (DH/T)th) -> (DH/T)th/1
  HPT Map lookup Table Efficency/1(HPT Ettath) -> etath/1

== system EngineModel_scaled_27_7_2016_with_new_maps/Double spool TFE CF6-50 steady state modeling (BOING 747-200)/Error Due to Vs/Error Due To Dv1/HPT/enthalpy_MAPS/Nch_Nth ==
  Tt4 : Inport
  Tt2.5 : Inport  Port=2
  Nch : Inport  Port=3
  (To)Ref : Constant  Value=288
  (theta4)d : Constant  Value=1.1018
  Display5 : Display
  Product3 : Product  Inputs=***  SaturateOnIntegerOverflow=on  OutDataTypeStr=Inherit: Same as first input
  Product4 : Product  Inputs=*/  SaturateOnIntegerOverflow=on  OutDataTypeStr=Inherit: Same as first input
  Product6 : Product  Inputs=*/  SaturateOnIntegerOverflow=on  OutDataTypeStr=Inherit: Same as first input
  Product7 : Product  Inputs=*/  SaturateOnIntegerOverflow=on  OutDataTypeStr=Inherit: Same as first input
  Sqrt1 : Sqrt  SaturateOnIntegerOverflow=on
  Sqrt2 : Sqrt  SaturateOnIntegerOverflow=on
  const. : Constant  Value=100
  Nth : Outport
  wires:
  Product7/1 -> Product3/1
  (To)Ref/1 -> Product4/2
  Sqrt1/1 -> Product7/2
  const./1 -> Product7/1
  Product3/1 -> Nth/1, Display5/1
  Tt4/1 -> Sqrt1/1
  Tt2.5/1 -> Product4/1
  Product4/1 -> Sqrt2/1
  (theta4)d/1 -> Product6/2
  Product6/1 -> Product3/2
  Sqrt2/1 -> Product6/1
  Nch/1 -> Product3/3

== system EngineModel_scaled_27_7_2016_with_new_maps/Double spool TFE CF6-50 steady state modeling (BOING 747-200)/Error Due to Vs/Error Due To Dv1/LPC/Adiabatic compression/isentropic compression ==
  Tt13 : Inport
  Prcl : Inport  Port=2
  P13 : Inport  Port=3
  Ht13 : Inport  Port=4
  S13 : Inport  Port=5
  etacl : Inport  Port=6
  Demux : Demux
      settings: DisplayOption=none
  Interpreted MATLAB Function : MATLABFcn  MATLABFcn=Adiabatic_compression_LPC(u(1),u(2),u(3),u(4),u(5),u(6))  OutputDimensions=4
  Mux : Mux  Inputs=6
      settings: DisplayOption=signals
  S25 : Outport
  Tt25 : Outport  Port=2
  Pt25 : Outport  Port=3
  Ht25 : Outport  Port=4
  wires:
  Tt13/1 -> Mux/1
  Demux/2 -> Pt25/1
  Interpreted MATLAB Function/1 -> Demux/1
  Demux/1 -> Tt25/1
  Mux/1 -> Interpreted MATLAB Function/1
  P13/1 -> Mux/3
  Prcl/1 -> Mux/2
  Ht13/1 -> Mux/4
  S13/1 -> Mux/5
  Demux/3 -> S25/1
  etacl/1 -> Mux/6
  Demux/4 -> Ht25/1

== system EngineModel_scaled_27_7_2016_with_new_maps/Double spool TFE CF6-50 steady state modeling (BOING 747-200)/Error Due to Vs/Error Due To Dv1/LPC/LPC Map/If condition Zcl ==
  Zcli : Inport
  Demux : Demux  Outputs=1
      settings: DisplayOption=none
  Interpreted MATLAB Function : MATLABFcn  MATLABFcn=if_Z(u(1))  OutputDimensions=1
  Mux : Mux  Inputs=1
      settings: DisplayOption=signals
  Zcl : Outport
  wires:
  Interpreted MATLAB Function/1 -> Demux/1
  Mux/1 -> Interpreted MATLAB Function/1
  Demux/1 -> Zcl/1
  Zcli/1 -> Mux/1

== system EngineModel_scaled_27_7_2016_with_new_maps/Double spool TFE CF6-50 steady state modeling (BOING 747-200)/Error Due to Vs/Error Due To Dv1/LPC/LPC Map/LPC Map Lookuptable efficiency ==
  corr Speed Ncl : Inport
  Zcl : Inport  Port=2
  3D fanmap Lookup Table : Lookup_n-D  NumberOfTableDimensions=3  BreakpointsForDimension1=[0.3,0.4,0.5,0.6,0.7,0.8,0.9,1.0,1.1,1.2]  BreakpointsForDimension2=[1,2,3]  BreakpointsForDimension3=[0,0.1,0.2,0.3,0.4,0.5,0.6,0.7,0.8,0.9,1]  IndexSearchMethod=Linear search  Table=LPCompmap_2  InterpMethod=Cubic spline  ExtrapMethod=Cubic spline  OutDataTypeStr=double  RndMeth=Simplest
      settings: InputPortMap=u0,u1,u2
  Constant1 : Constant  Value=3
  Display : Display
  etacl : Outport
  wires:
  corr Speed Ncl/1 -> 3D fanmap Lookup Table/1
  Constant1/1 -> 3D fanmap Lookup Table/2
  3D fanmap Lookup Table/1 -> etacl/1, Display/1
  Zcl/1 -> 3D fanmap Lookup Table/3

== system EngineModel_scaled_27_7_2016_with_new_maps/Double spool TFE CF6-50 steady state modeling (BOING 747-200)/Error Due to Vs/Error Due To Dv1/LPC/LPC Map/LPC Map Lookuptable massflow ==
  corr Speed Ncl : Inport
  Zcl : Inport  Port=2
  3D fanmap Lookup Table : Lookup_n-D  NumberOfTableDimensions=3  BreakpointsForDimension1=[0.3,0.4,0.5,0.6,0.7,0.8,0.9,1.0,1.1,1.2]  BreakpointsForDimension2=[1,2,3]  BreakpointsForDimension3=[0,0.1,0.2,0.3,0.4,0.5,0.6,0.7,0.8,0.9,1]  IndexSearchMethod=Linear search  Table=LPCompmap_2  InterpMethod=Cubic spline  ExtrapMethod=Cubic spline  OutDataTypeStr=double  RndMeth=Simplest
      settings: InputPortMap=u0,u1,u2
  Constant1 : Constant  Value=2
  Display : Display
  " MFPcl" : Outport
  wires:
  corr Speed Ncl/1 -> 3D fanmap Lookup Table/1
  Constant1/1 -> 3D fanmap Lookup Table/2
  3D fanmap Lookup Table/1 -> " MFPcl"/1, Display/1
  Zcl/1 -> 3D fanmap Lookup Table/3

== system EngineModel_scaled_27_7_2016_with_new_maps/Double spool TFE CF6-50 steady state modeling (BOING 747-200)/Error Due to Vs/Error Due To Dv1/LPC/LPC Map/LPC Map Lookuptable pressure ratio ==
  corr Speed Ncl : Inport
  Zcl : Inport  Port=2
  3D fanmap Lookup Table : Lookup_n-D  NumberOfTableDimensions=3  BreakpointsForDimension1=[0.3,0.4,0.5,0.6,0.7,0.8,0.9,1.0,1.1,1.2]  BreakpointsForDimension2=[1,2,3]  BreakpointsForDimension3=[0,0.1,0.2,0.3,0.4,0.5,0.6,0.7,0.8,0.9,1]  IndexSearchMethod=Linear search  Table=LPCompmap_2  InterpMethod=Cubic spline  ExtrapMethod=Cubic spline  OutDataTypeStr=double  RndMeth=Simplest
      settings: InputPortMap=u0,u1,u2
  Constant1 : Constant
  Display : Display
  " Prcl" : Outport
  wires:
  Zcl/1 -> 3D fanmap Lookup Table/3
  3D fanmap Lookup Table/1 -> Display/1, " Prcl"/1
  Constant1/1 -> 3D fanmap Lookup Table/2
  corr Speed Ncl/1 -> 3D fanmap Lookup Table/1

== system EngineModel_scaled_27_7_2016_with_new_maps/Double spool TFE CF6-50 steady state modeling (BOING 747-200)/Error Due to Vs/Error Due To Dv1/LPT/enthalpy_MAPS/LPT map ==
  Ntl : Inport
  TFtl : Inport  Port=2
  LPT Map lookup Table (DH/T) : Subsystem
  LPT Map lookup Table Efficency : Subsystem
  (DH/T)tl : Outport
  etatl : Outport  Port=2
  wires:
  Ntl/1 -> LPT Map lookup Table Efficency/1(corr speed Ntl), LPT Map lookup Table (DH/T)/1(corr speed Ntl)
  TFtl/1 -> LPT Map lookup Table Efficency/2(TFtl), LPT Map lookup Table (DH/T)/2(TFtl)
  LPT Map lookup Table (DH/T)/1(LPT (DH/T)tl) -> (DH/T)tl/1
  LPT Map lookup Table Efficency/1(HPT Ettatl) -> etatl/1

== system EngineModel_scaled_27_7_2016_with_new_maps/Double spool TFE CF6-50 steady state modeling (BOING 747-200)/Error Due to Vs/Error Due To Dv1/LPT/enthalpy_MAPS/Nch_Nth ==
  Tt45 : Inport
  Tt2 : Inport  Port=2
  Ncf : Inport  Port=3
  (To)Ref : Constant  Value=288
  (theta2)d : Constant  Value=0.9532186
  Display5 : Display
  Product3 : Product  Inputs=**  SaturateOnIntegerOverflow=on  OutDataTypeStr=Inherit: Same as first input
  Product4 : Product  Inputs=*/  SaturateOnIntegerOverflow=on  OutDataTypeStr=Inherit: Same as first input
  Product6 : Product  Inputs=*/  SaturateOnIntegerOverflow=on  OutDataTypeStr=Inherit: Same as first input
  Product7 : Product  Inputs=*/  SaturateOnIntegerOverflow=on  OutDataTypeStr=Inherit: Same as first input
  Product8 : Product  Inputs=**  SaturateOnIntegerOverflow=on  OutDataTypeStr=Inherit: Same as first input
  Sqrt1 : Sqrt  SaturateOnIntegerOverflow=on
  Sqrt2 : Sqrt  SaturateOnIntegerOverflow=on
  const. : Constant  Value=100
  Ntl : Outport
  wires:
  Product8/1 -> Product3/1
  (To)Ref/1 -> Product4/2
  Product7/1 -> Product8/1
  Sqrt1/1 -> Product7/2
  const./1 -> Product7/1
  Product3/1 -> Display5/1, Ntl/1
  Ncf/1 -> Product3/2
  Tt45/1 -> Sqrt1/1
  Tt2/1 -> Product4/1
  Product4/1 -> Sqrt2/1
  (theta2)d/1 -> Product6/2
  Product6/1 -> Product8/2
  Sqrt2/1 -> Product6/1

== system EngineModel_scaled_27_7_2016_with_new_maps/Double spool TFE CF6-50 steady state modeling (BOING 747-200)/Error Due to Vs/Error Due To Dv1/Ram/If condition PRF/If Action Subsystem ==
  In1 : Inport
  Action Port : ActionPort  ActionPortLabel=if(u1 <1)
  Out1 : Outport
  wires:
  In1/1 -> Out1/1

== system EngineModel_scaled_27_7_2016_with_new_maps/Double spool TFE CF6-50 steady state modeling (BOING 747-200)/Error Due to Vs/Error Due To Dv1/Ram/If condition PRF/If Action Subsystem1 ==
  In1 : Inport
  Action Port : ActionPort  ActionPortLabel=else
  Out1 : Outport
  wires:
  In1/1 -> Out1/1
